simulink model "ST5B_feedback"  (R2020a)
settings: Solver=FixedStepAuto  StartTime=0.0  StopTime=4.5  FixedStep=0.005  RelTol=1e-3
undefined symbols (not defined in the file): Efd0, Kc, Kr, T1, Tr, Vinit, VR0, Vrmax, Vrmin, XadIfd
libraries: eeGeneralControl x5, simulink x1
settings Model: Creator=meagh  LastModifiedBy=meagh

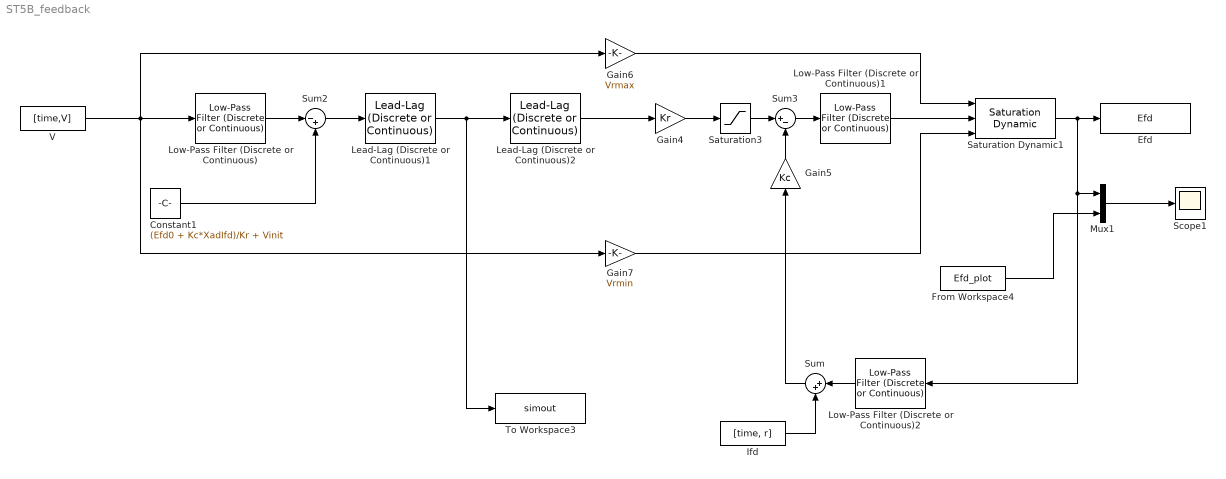
== system ST5B_feedback ==
  Constant1 : Constant  Value=(Efd0 + Kc*XadIfd)/Kr + Vinit
  Efd : ToWorkspace  VariableName=Efd  SaveFormat=Timeseries  SampleTime=-1
  From Workspace4 : FromWorkspace  VariableName=Efd_plot
  Gain4 : Gain  Gain=Kr
  Gain5 : Gain  Gain=Kc
  Gain6 : Gain  Gain=Vrmax
  Gain7 : Gain  Gain=Vrmin
  Ifd : FromWorkspace  VariableName=[time, r]
  Lead-Lag (Discrete or Continuous)1 : eeGeneralControl/Lead-Lag (Discrete or Continuous)  T1=Tb1  T2=Tc1  B=Vrmax/Kr  A=Vrmin/Kr  init_option=Inherited from block input  x0=VR0/Kr  Ts=0
      settings: SourceProductBaseCode=PS
  Lead-Lag (Discrete or Continuous)2 : eeGeneralControl/Lead-Lag (Discrete or Continuous)  T1=Tb2  T2=Tc2  B=Vrmax/Kr  A=Vrmin/Kr  init_option=Inherited from block input  x0=VR0/Kr  Ts=0
      settings: SourceProductBaseCode=PS
  Low-Pass Filter (Discrete or Continuous) : eeGeneralControl/Low-Pass Filter (Discrete or Continuous)  K=1  T=Tr  B=inf  A=-inf  init_option=Inherited from block input  x0=0  Ts=0
  Low-Pass Filter (Discrete or Continuous)1 : eeGeneralControl/Low-Pass Filter (Discrete or Continuous)  K=1  T=T1  B=inf  A=-inf  init_option=Inherited from block input  x0=0  Ts=0
  Low-Pass Filter (Discrete or Continuous)2 : eeGeneralControl/Low-Pass Filter (Discrete or Continuous)  K=1  T=1  B=inf  A=-inf  init_option=Inherited from block input  x0=0  Ts=0
  Mux1 : Mux  Inputs=2
  Saturation Dynamic1 : simulink/Discontinuities/Saturation Dynamic  OutMin=[]  OutMax=[]  OutDataTypeStr=Inherit: Same as second input  OutDataType=fixdt(1, 16)  OutScaling=2^-10  DoSatur=off
  Saturation3 : Saturate  UpperLimit=Vrmax  LowerLimit=Vrmin  LinearizeAsGain=off
  Scope1 : Scope
  Sum : Sum  Inputs=|++
  Sum2 : Sum  Inputs=|-+
  Sum3 : Sum  Inputs=|+-
  To Workspace3 : ToWorkspace  VariableName=simout  SaveFormat=Timeseries  SampleTime=-1
  V : FromWorkspace  VariableName=[time,V]
  wires:
  Constant1/1 -> Sum2/2
  Gain7/1 -> Saturation Dynamic1/3
  From Workspace4/1 -> Mux1/2
  Mux1/1 -> Scope1/1
  Saturation Dynamic1/1 -> Low-Pass Filter (Discrete or Continuous)2/1, Mux1/1, Efd/1
  Sum3/1 -> Low-Pass Filter (Discrete or Continuous)1/1
  Gain6/1 -> Saturation Dynamic1/1
  Saturation3/1 -> Sum3/1
  Gain5/1 -> Sum3/2
  V/1 -> Low-Pass Filter (Discrete or Continuous)/1, Gain7/1, Gain6/1
  Sum2/1 -> Lead-Lag (Discrete or Continuous)1/1
  Low-Pass Filter (Discrete or Continuous)/1 -> Sum2/1
  Low-Pass Filter (Discrete or Continuous)1/1 -> Saturation Dynamic1/2
  Gain4/1 -> Saturation3/1
  Lead-Lag (Discrete or Continuous)1/1 -> To Workspace3/1, Lead-Lag (Discrete or Continuous)2/1
  Lead-Lag (Discrete or Continuous)2/1 -> Gain4/1
  Sum/1 -> Gain5/1
  Low-Pass Filter (Discrete or Continuous)2/1 -> Sum/1
  Ifd/1 -> Sum/2
